simulink model "SCG007C_TC_Development_r01"  (R2017b)
settings: Solver=VariableStepAuto  StartTime=0.0  StopTime=10.0  RelTol=1e-3
values from neighbouring files (symbols this model uses):
  MP_SLIP_val = [ ... (first row only)    [Calibration_r01_v01.m]
  MP_SLIP_x1 = [0.000 0.500 0.750 1.000 1.250 1.500 1.750 2.000 2.500]./2.5.*100    [Calibration_r01_v01.m]
  MP_SLIP_x2 = [0	1	2	3	4	5	6	7	8	9	10	11	12]    [Calibration_r01_v01.m]
  MP_SLIPIP_DSLIP_val = [ ... (first row only)    [Calibration_r01_v01.m]
  MP_SLIPIP_DSLIP_x1 = [0.0 20.0 40.0 60.0 70.0 80.0 90.0 100.0 110.0 120.0 140.0]    [Calibration_r01_v01.m]
  MP_SLIPIP_DSLIP_x2 = [-4.0 -2.0 -1.0 -0.6 0.0 0.1 0.5 3.0 5.0]    [Calibration_r01_v01.m]
  MP_SLIPPP_DSLIP_val = [ ... (first row only)    [Calibration_r01_v01.m]
  MP_SLIPPP_DSLIP_x1 = [0.0 20.0 40.0 60.0 70.0 80.0 90.0 100.0 110.0 120.0 140.0]    [Calibration_r01_v01.m]
  MP_SLIPPP_DSLIP_x2 = [-4.0 -2.0 -1.0 -0.6 0.0 0.1 0.5 3.0 5.0]    [Calibration_r01_v01.m]
undefined symbols (not defined in the file or in its folder): Engine, Standard_Input_Bus, TCS, vicrt_initcallback, vicrt_initmexcallback, vicrt_simulationmanager
libraries: simulink x7, simulink_extras x1
(part 1 of 5)
settings Model: Creator=Stefano.Rapisarda  LastModifiedBy=Stefano.Rapisarda

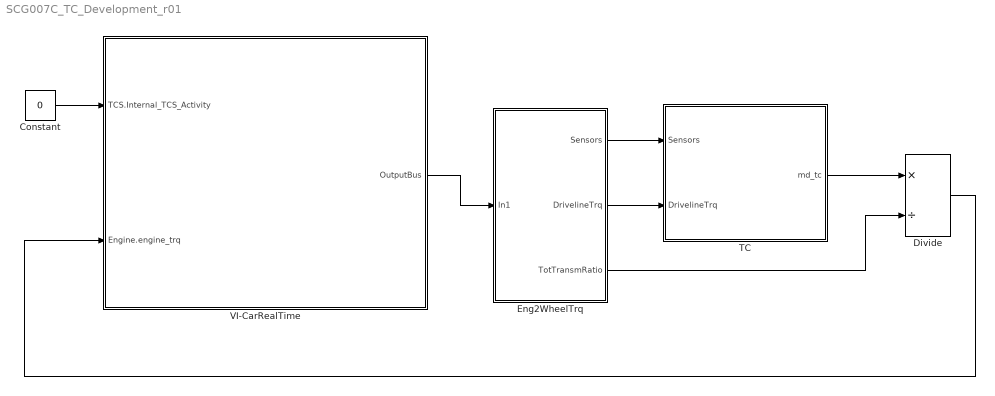
== system SCG007C_TC_Development_r01 ==
  Constant : Constant  Value=0
  Divide : Product  Inputs=*/
  Eng2WheelTrq : Subsystem
  TC : Subsystem
  VI-CarRealTime : Subsystem  InitFcn=vicrt_simulationmanager(0);
      mask help: Full VI-CarRealTime mex integrated with IO Bus
      settings: CopyFcn=set_param(gcb, 'LinkStatus', 'none');  ModelCloseFcn=vicrt_simulationmanager(2);  OpenFcn=vicrt_simulationmanager(1);
      mask Display: image(imread('vehicle.jpg'));color('red');port_label('input',1,'TCS.Internal_TCS_Activity');port_label('input',2,'Engine.engine_trq');port_label('output',1,'OutputBus');
  wires:
  VI-CarRealTime/1(OutputBus) -> Eng2WheelTrq/1(In1)
  TC/1(md_tc) -> Divide/1
  Constant/1 -> VI-CarRealTime/1(TCS.Internal_TCS_Activity)
  Divide/1 -> VI-CarRealTime/2(Engine.engine_trq)
  Eng2WheelTrq/1(Sensors) -> TC/1(Sensors)
  Eng2WheelTrq/2(DrivelineTrq) -> TC/2(DrivelineTrq)
  Eng2WheelTrq/3(TotTransmRatio) -> Divide/2

== system SCG007C_TC_Development_r01/Eng2WheelTrq ==
  In1 : Inport
  Bus Creator : BusCreator  Inputs=2
  Bus Selector : BusSelector  OutputSignals=engine:Max_Engine_torque,engine:Min_engine_torque,transmission:ratio
  Product : Product
  Product1 : Product
  Product2 : Product
  RearDiffRatio : Constant  Value=3.02
  Sensors : Outport
  DrivelineTrq : Outport  Port=2
  TotTransmRatio : Outport  Port=3
  wires:
  In1/1 -> Sensors/1, Bus Selector/1
  Bus Selector/3 -> Product/1  "<transmission:ratio>"
  RearDiffRatio/1 -> Product/2
  Bus Selector/2 -> Product1/1  "<engine:Min_engine_torque>"
  Bus Selector/1 -> Product2/1  "<engine:Max_Engine_torque>"
  Product/1 -> TotTransmRatio/1, Product1/2, Product2/2
  Product2/1 -> Bus Creator/1  "MaxDrivelineTrq"
  Product1/1 -> Bus Creator/2  "MinDrivelineTrq"
  Bus Creator/1 -> DrivelineTrq/1

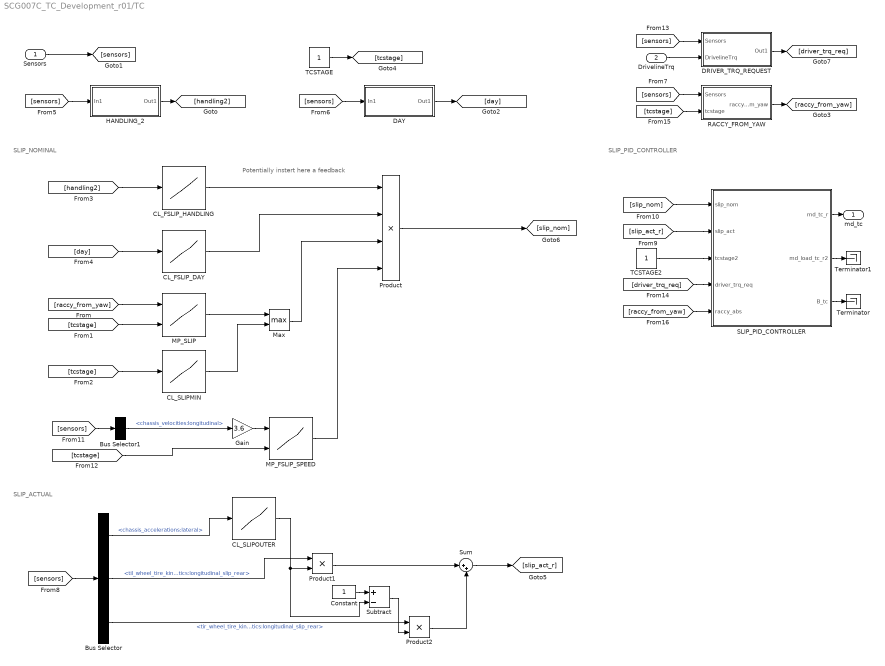
== system SCG007C_TC_Development_r01/TC ==
  note: SLIP_PID_CONTROLLER
  note: Potentially instert here a feedback
  note: SLIP_ACTUAL
  note: SLIP_NOMINAL
  Sensors : Inport
  DrivelineTrq : Inport  Port=2
  Bus Selector : BusSelector  OutputSignals=chassis_accelerations:lateral,til_wheel_tire_kinematics:longitudinal_slip_rear,tir_wheel_tire_kinematics:longitudinal_slip_rear
  Bus Selector1 : BusSelector  OutputSignals=chassis_velocities:longitudinal
  CL_FSLIP_DAY : Lookup_n-D  NumberOfTableDimensions=1  BreakpointsForDimension1=[-1,0,1]  Table=[1,1,1]  InternalRulePriority=Speed  RndMeth=Simplest  InputSameDT=on
  CL_FSLIP_HANDLING : Lookup_n-D  NumberOfTableDimensions=1  BreakpointsForDimension1=[-1,0,1]  Table=[1,1,1]  InternalRulePriority=Speed  RndMeth=Simplest  InputSameDT=on
  CL_SLIPMIN : Lookup_n-D  NumberOfTableDimensions=1  BreakpointsForDimension1=[1,2,3]  Table=[2,2,2]  InternalRulePriority=Speed  RndMeth=Simplest  InputSameDT=on
  CL_SLIPOUTER : Lookup_n-D  NumberOfTableDimensions=1  BreakpointsForDimension1=[-3,-2,-1,0,1,2,3]  Table=[0.8,0.7,0.6,0.5,0.6,0.7,0.8]  InternalRulePriority=Speed  RndMeth=Simplest  InputSameDT=on
  Constant : Constant
  DAY : Subsystem
  DRIVER_TRQ_REQUEST : Subsystem
  Gain : Gain  Gain=3.6
  HANDLING_2 : Subsystem
  MP_FSLIP_SPEED : Lookup_n-D  LookupTableObject=''  BreakpointsForDimension1=[0,500]  BreakpointsForDimension2=[1,2,3]  BreakpointsForDimension1FirstPoint=10  BreakpointsForDimension2FirstPoint=10  BreakpointsForDimension1Spacing=12  BreakpointsForDimension2Spacing=12  IndexSearchMethod=Evenly spaced points  Table=[1 1 1;1 1 1]  InterpMethod=Flat  DiagnosticForOutOfRangeInput=Error  InternalRulePriority=Speed  RndMeth=Simplest  InputSameDT=on
  MP_SLIP : Lookup_n-D  LookupTableObject=''  BreakpointsForDimension1=MP_SLIP_x1  BreakpointsForDimension2=MP_SLIP_x2  BreakpointsForDimension1FirstPoint=10  BreakpointsForDimension2FirstPoint=10  BreakpointsForDimension1Spacing=12  BreakpointsForDimension2Spacing=12  IndexSearchMethod=Evenly spaced points  Table=MP_SLIP_val  InterpMethod=Flat  DiagnosticForOutOfRangeInput=Error  InternalRulePriority=Speed  RndMeth=Simplest  InputSameDT=on
  Max : MinMax  Function=max  Inputs=2
  Product : Product  Inputs=4
  Product1 : Product
  Product2 : Product
  RACCY_FROM_YAW : Subsystem
  SLIP_PID_CONTROLLER : Subsystem
  Subtract : Sum  Inputs=+-
  Sum : Sum  Inputs=|++
  TCSTAGE : Constant
  TCSTAGE2 : Constant
  Terminator : Terminator
  Terminator1 : Terminator
  md_tc : Outport
  wires:
  [raccy_from_yaw] -> MP_SLIP/1
  [tcstage] -> MP_SLIP/2
  [tcstage] -> CL_SLIPMIN/1
  [handling2] -> CL_FSLIP_HANDLING/1
  [day] -> CL_FSLIP_DAY/1
  MP_SLIP/1 -> Max/1
  CL_SLIPMIN/1 -> Max/2
  CL_FSLIP_HANDLING/1 -> Product/1
  CL_FSLIP_DAY/1 -> Product/2
  Max/1 -> Product/3
  Sensors/1 -> [sensors]
  HANDLING_2/1(Out1) -> [handling2]
  [sensors] -> HANDLING_2/1(In1)
  [sensors] -> DAY/1(In1)
  DAY/1(Out1) -> [day]
  [sensors] -> RACCY_FROM_YAW/1(Sensors)
  RACCY_FROM_YAW/1(raccy_from_yaw) -> [raccy_from_yaw]
  TCSTAGE/1 -> [tcstage]
  [sensors] -> Bus Selector/1
  Bus Selector/2 -> Product1/1  "<til_wheel_tire_kinematics:longitudinal_slip_rear>"
  Bus Selector/1 -> CL_SLIPOUTER/1  "<chassis_accelerations:lateral>"
  Constant/1 -> Subtract/1
  CL_SLIPOUTER/1 -> Subtract/2, Product1/2
  Bus Selector/3 -> Product2/1  "<tir_wheel_tire_kinematics:longitudinal_slip_rear>"
  Subtract/1 -> Product2/2
  Product1/1 -> Sum/1
  Product2/1 -> Sum/2
  Sum/1 -> [slip_act_r]
  Product/1 -> [slip_nom]
  [slip_nom] -> SLIP_PID_CONTROLLER/1(slip_nom)
  [slip_act_r] -> SLIP_PID_CONTROLLER/2(slip_act)
  SLIP_PID_CONTROLLER/1(md_tc_r) -> md_tc/1
  MP_FSLIP_SPEED/1 -> Product/4
  [sensors] -> Bus Selector1/1
  Bus Selector1/1 -> Gain/1  "<chassis_velocities:longitudinal>"
  [tcstage] -> MP_FSLIP_SPEED/2
  SLIP_PID_CONTROLLER/3(B_tc) -> Terminator/1
  SLIP_PID_CONTROLLER/2(md_load_tc_r2) -> Terminator1/1
  TCSTAGE2/1 -> SLIP_PID_CONTROLLER/3(tcstage2)
  [sensors] -> DRIVER_TRQ_REQUEST/1(Sensors)
  DRIVER_TRQ_REQUEST/1(Out1) -> [driver_trq_req]
  [driver_trq_req] -> SLIP_PID_CONTROLLER/4(driver_trq_req)
  Gain/1 -> MP_FSLIP_SPEED/1
  [tcstage] -> RACCY_FROM_YAW/2(tcstage)
  DrivelineTrq/1 -> DRIVER_TRQ_REQUEST/2(DrivelineTrq)
  [raccy_from_yaw] -> SLIP_PID_CONTROLLER/5(raccy_abs)

== system SCG007C_TC_Development_r01/VI-CarRealTime ==
  TCS.Internal_TCS_Activity : Inport
  Engine.engine_trq : Inport  Port=2
  Input_Bus : Subsystem  LoadFcn=vicrt_initcallback(gcb);
      settings: CopyFcn=vicrt_initcallback(gcb);
  Output_Bus : Subsystem  Description=Outputs
      settings: CopyFcn=%set_param(gcb, 'LinkStatus', 'none')
  vicrt_mex Standard : Subsystem  mask{vicrt_inputfile='D:\VI-Grade_WD\SCG007C_2\SCG007C_R07_500kW_BaseSetupSiff_Coasting_send_svm.xml', vicrt_outprefix='', intStep=0.001, AniFlag=off, inpPortDim=378, outPortDim=1516, NoDirectFeedthrough=on}
      mask prompts: vicrt_inputfile "VI-CarRealtime input file"; vicrt_outprefix "VI-CarRealTime output prefix"; intStep "Integration step"; AniFlag "live animation"; inpPortDim "input port dimension"; outPortDim "output port dimension"; NoDirectFeedthrough "Direct Feedthrough Off"
      mask init:
      | custDriv=[1,1,1];
      settings: CopyFcn=set_param(gcb, 'LinkStatus', 'none')
  OutputBus : Outport
  wires:
  vicrt_mex Standard/1(Out1) -> Output_Bus/1(Outputs)
  Input_Bus/1(vicrt input) -> vicrt_mex Standard/1(In1)
  TCS.Internal_TCS_Activity/1 -> Input_Bus/1(TCS.Internal_TCS_Activity)
  Engine.engine_trq/1 -> Input_Bus/2(Engine.engine_trq)
  Output_Bus/1(OutputBus) -> OutputBus/1

== system SCG007C_TC_Development_r01/TC/DAY ==
  In1 : Inport
  Constant : Constant  Value=0
  Terminator : Terminator
  Out1 : Outport
  wires:
  Constant/1 -> Out1/1
  In1/1 -> Terminator/1

== system SCG007C_TC_Development_r01/TC/DRIVER_TRQ_REQUEST ==
  Sensors : Inport
  DrivelineTrq : Inport  Port=2
  Add : Sum
  Bus Selector : BusSelector  OutputSignals=engine:Max_Engine_torque,engine:Min_engine_torque,driver_demands:throttle
  Bus Selector1 : BusSelector  OutputSignals=MaxDrivelineTrq,MinDrivelineTrq
  Product : Product
  Subtract : Sum  Inputs=+-
  Terminator : Terminator
  Terminator2 : Terminator
  Out1 : Outport
  wires:
  Sensors/1 -> Bus Selector/1
  Subtract/1 -> Product/1
  Product/1 -> Add/1
  Add/1 -> Out1/1
  Bus Selector/2 -> Terminator/1  "<engine:Min_engine_torque>"
  Bus Selector/3 -> Product/2  "<driver_demands:throttle>"
  Bus Selector/1 -> Terminator2/1  "<engine:Max_Engine_torque>"
  DrivelineTrq/1 -> Bus Selector1/1
  Bus Selector1/1 -> Subtract/1  "<MaxDrivelineTrq>"
  Bus Selector1/2 -> Add/2, Subtract/2  "<MinDrivelineTrq>"

== system SCG007C_TC_Development_r01/TC/HANDLING_2 ==
  In1 : Inport
  Constant : Constant  Value=0
  Terminator : Terminator
  Out1 : Outport
  wires:
  In1/1 -> Terminator/1
  Constant/1 -> Out1/1

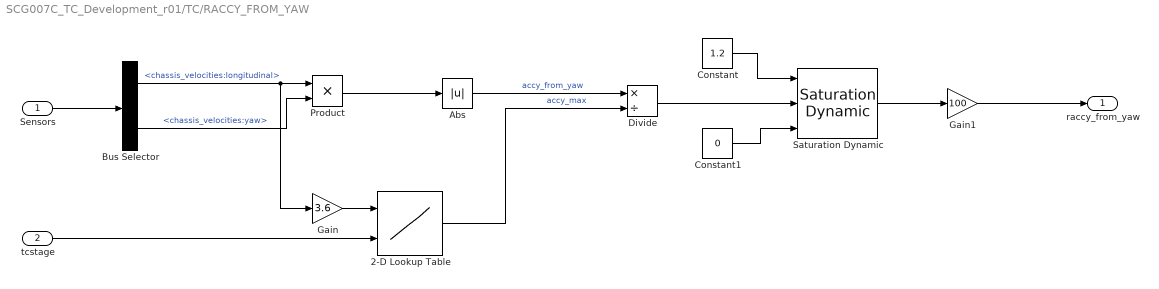
== system SCG007C_TC_Development_r01/TC/RACCY_FROM_YAW ==
  Sensors : Inport
  tcstage : Inport  Port=2
  2-D Lookup Table : Lookup_n-D  BreakpointsForDimension1=[1:3]  BreakpointsForDimension2=[1:3]  InternalRulePriority=Speed  RndMeth=Simplest  InputSameDT=on
  Abs : Abs
  Bus Selector : BusSelector  OutputSignals=chassis_velocities:longitudinal,chassis_velocities:yaw
  Constant : Constant  Value=1.2
  Constant1 : Constant  Value=0
  Divide : Product  Inputs=*/
  Gain : Gain  Gain=3.6
  Gain1 : Gain  Gain=100
  Product : Product
  Saturation Dynamic : simulink/Discontinuities/Saturation Dynamic  OutMin=[]  OutMax=[]  OutDataTypeStr=Inherit: Same as second input  OutDataType=fixdt(1, 16)  OutScaling=2^-10  DoSatur=off
  raccy_from_yaw : Outport
  wires:
  Sensors/1 -> Bus Selector/1
  Bus Selector/1 -> Gain/1, Product/1  "<chassis_velocities:longitudinal>"
  Bus Selector/2 -> Product/2  "<chassis_velocities:yaw>"
  Product/1 -> Abs/1
  Abs/1 -> Divide/1  "accy_from_yaw"
  2-D Lookup Table/1 -> Divide/2  "accy_max"
  Divide/1 -> Saturation Dynamic/2
  Constant/1 -> Saturation Dynamic/1
  Constant1/1 -> Saturation Dynamic/3
  Saturation Dynamic/1 -> Gain1/1
  Gain/1 -> 2-D Lookup Table/1
  tcstage/1 -> 2-D Lookup Table/2
  Gain1/1 -> raccy_from_yaw/1

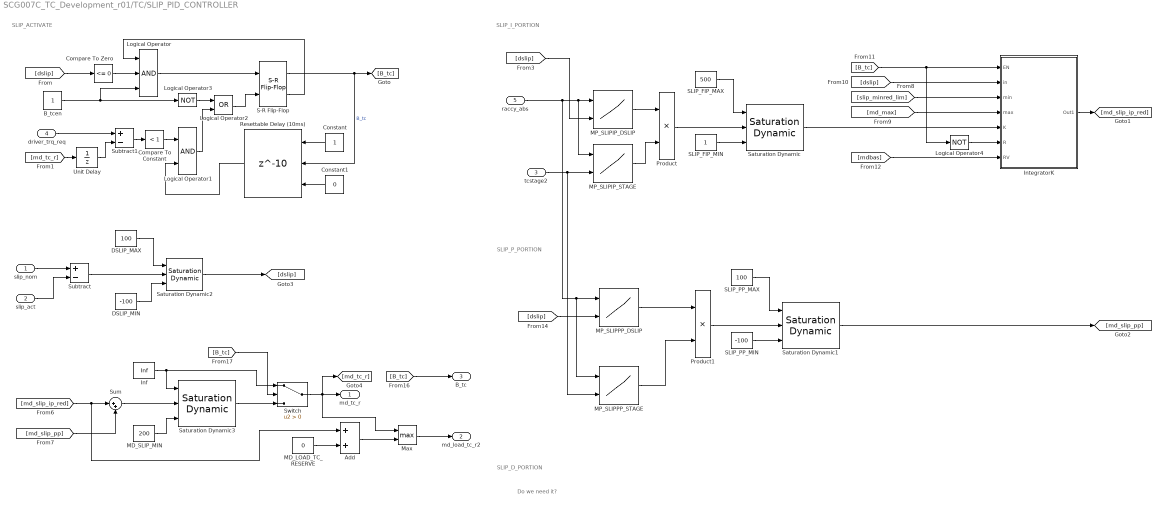
== system SCG007C_TC_Development_r01/TC/SLIP_PID_CONTROLLER ==
  note: Do we need it?
  note: SLIP_I_PORTION
  note: SLIP_ACTIVATE
  note: SLIP_P_PORTION
  note: SLIP_D_PORTION
  slip_nom : Inport
  slip_act : Inport  Port=2
  tcstage2 : Inport  Port=3
  driver_trq_req : Inport  Port=4
  raccy_abs : Inport  Port=5
  Add : Sum
  B_tcen : Constant
  Compare To Constant : simulink/Logic and Bit Operations/Compare To Constant  relop=<  const=1  OutDataTypeStr=boolean
  Compare To Zero : simulink/Logic and Bit Operations/Compare To Zero  relop=<=  OutDataTypeStr=boolean
  Constant : Constant
  Constant1 : Constant  Value=0
  DSLIP_MAX : Constant  Value=100
  DSLIP_MIN : Constant  Value=-100
  Inf : Constant  Value=Inf
  IntegratorK : Subsystem
  Logical Operator : Logic  Inputs=3  AllPortsSameDT=off  OutDataTypeStr=boolean
  Logical Operator1 : Logic  AllPortsSameDT=off  OutDataTypeStr=boolean
  Logical Operator2 : Logic  Operator=OR  AllPortsSameDT=off  OutDataTypeStr=boolean
  Logical Operator3 : Logic  Operator=NOT  AllPortsSameDT=off  OutDataTypeStr=boolean
  Logical Operator4 : Logic  Operator=NOT  AllPortsSameDT=off  OutDataTypeStr=boolean
  MD_LOAD_TC_RESERVE : Constant  Value=0
  MD_SLIP_MIN : Constant  Value=200
  MP_SLIPIP_DSLIP : Lookup_n-D  BreakpointsForDimension1=MP_SLIPIP_DSLIP_x1  BreakpointsForDimension2=MP_SLIPIP_DSLIP_x2  Table=MP_SLIPIP_DSLIP_val  InternalRulePriority=Speed  RndMeth=Simplest  InputSameDT=on
  MP_SLIPIP_STAGE : Lookup_n-D  BreakpointsForDimension1=[0,20,40,60,70,80,90,100,110,120,140]  BreakpointsForDimension2=[0,1]  Table=reshape([1,1,1,1,1,1,1,1,1,1,1,1,1,1,1,1,1,1,1,1,1,1],11,2)  InternalRulePriority=Speed  RndMeth=Simplest  InputSameDT=on
  MP_SLIPPP_DSLIP : Lookup_n-D  BreakpointsForDimension1=MP_SLIPPP_DSLIP_x1  BreakpointsForDimension2=MP_SLIPPP_DSLIP_x2  Table=MP_SLIPPP_DSLIP_val  InternalRulePriority=Speed  RndMeth=Simplest  InputSameDT=on
  MP_SLIPPP_STAGE : Lookup_n-D  BreakpointsForDimension1=[0,20,40,60,70,80,90,100,110,120,140]  BreakpointsForDimension2=[0,1]  Table=reshape([1,1,1,1,1,1,1,1,1,1,1,1,1,1,1,1,1,1,1,1,1,1],11,2)  InternalRulePriority=Speed  RndMeth=Simplest  InputSameDT=on
  Max : MinMax  Function=max  Inputs=2
  Product : Product
  Product1 : Product
  Resettable Delay (10ms) : Delay  DelayLength=10  InitialConditionSource=Input port  ExternalReset=Rising
      settings: InputPortMap=u0,r5,p4
  S-R Flip-Flop : simulink_extras/Flip Flops/S-R Flip-Flop  initial_condition=0
  SLIP_FIP_MAX : Constant  Value=500
  SLIP_FIP_MIN : Constant
  SLIP_PP_MAX : Constant  Value=100
  SLIP_PP_MIN : Constant  Value=-100
  Saturation Dynamic{,1..3} (4 alike) : simulink/Discontinuities/Saturation Dynamic  OutMin=[]  OutMax=[]  OutDataTypeStr=Inherit: Same as second input  OutDataType=fixdt(1, 16)  OutScaling=2^-10  DoSatur=off
  Subtract : Sum  Inputs=+-
  Subtract1 : Sum  Inputs=+-
  Sum : Sum  Inputs=|++
  Switch : Switch  Criteria=u2 > Threshold
  Unit Delay : UnitDelay  SampleTime=-1
  md_tc_r : Outport
  md_load_tc_r2 : Outport  Port=2
  B_tc : Outport  Port=3
  wires:
  [dslip] -> Compare To Zero/1
  Compare To Zero/1 -> Logical Operator/2
  S-R Flip-Flop/2 -> Logical Operator/1
  Logical Operator/1 -> S-R Flip-Flop/1
  B_tcen/1 -> Logical Operator/3, Logical Operator3/1
  Constant/1 -> Resettable Delay (10ms)/1
  Constant1/1 -> Resettable Delay (10ms)/3
  Resettable Delay (10ms)/1 -> Logical Operator1/2
  Logical Operator2/1 -> S-R Flip-Flop/2
  S-R Flip-Flop/1 -> [B_tc], Resettable Delay (10ms)/2  "B_tc"
  Logical Operator3/1 -> Logical Operator2/1
  Logical Operator1/1 -> Logical Operator2/2
  [dslip] -> MP_SLIPIP_DSLIP/2
  MP_SLIPIP_DSLIP/1 -> Product/1
  MP_SLIPIP_STAGE/1 -> Product/2
  Product/1 -> Saturation Dynamic/2
  SLIP_FIP_MAX/1 -> Saturation Dynamic/1
  SLIP_FIP_MIN/1 -> Saturation Dynamic/3
  [md_max] -> IntegratorK/4(max)
  [slip_minred_lim] -> IntegratorK/3(min)
  [dslip] -> IntegratorK/2(in)
  [B_tc] -> Logical Operator4/1, IntegratorK/1(EN)
  Saturation Dynamic/1 -> IntegratorK/5(K)
  Logical Operator4/1 -> IntegratorK/6(R)
  [mdbas] -> IntegratorK/7(RV)
  IntegratorK/1(Out1) -> [md_slip_ip_red]
  raccy_abs/1 -> MP_SLIPPP_STAGE/1, MP_SLIPPP_DSLIP/1, MP_SLIPIP_STAGE/1, MP_SLIPIP_DSLIP/1
  [dslip] -> MP_SLIPPP_DSLIP/2
  tcstage2/1 -> MP_SLIPPP_STAGE/2, MP_SLIPIP_STAGE/2
  MP_SLIPPP_DSLIP/1 -> Product1/1
  MP_SLIPPP_STAGE/1 -> Product1/2
  SLIP_PP_MIN/1 -> Saturation Dynamic1/3
  SLIP_PP_MAX/1 -> Saturation Dynamic1/1
  Product1/1 -> Saturation Dynamic1/2
  Saturation Dynamic1/1 -> [md_slip_pp]
  [B_tc] -> B_tc/1
  Subtract/1 -> Saturation Dynamic2/2
  slip_nom/1 -> Subtract/1
  slip_act/1 -> Subtract/2
  DSLIP_MIN/1 -> Saturation Dynamic2/3
  DSLIP_MAX/1 -> Saturation Dynamic2/1
  Saturation Dynamic2/1 -> [dslip]
  [md_slip_ip_red] -> Add/1, Sum/1
  [md_slip_pp] -> Sum/2
  Sum/1 -> Saturation Dynamic3/2
  MD_SLIP_MIN/1 -> Saturation Dynamic3/3
  Inf/1 -> Switch/1, Saturation Dynamic3/1
  Saturation Dynamic3/1 -> Switch/3
  [B_tc] -> Switch/2
  Switch/1 -> [md_tc_r], Max/1, md_tc_r/1
  Add/1 -> Max/2
  Max/1 -> md_load_tc_r2/1
  MD_LOAD_TC_RESERVE/1 -> Add/2
  [md_tc_r] -> Unit Delay/1
  driver_trq_req/1 -> Subtract1/1
  Unit Delay/1 -> Subtract1/2
  Subtract1/1 -> Compare To Constant/1
  Compare To Constant/1 -> Logical Operator1/1

== system SCG007C_TC_Development_r01/VI-CarRealTime/Input_Bus ==
  TCS.Internal_TCS_Activity : Inport
  Engine.engine_trq : Inport  Port=2
  Bus2Map : Subsystem
  Inputs : Subsystem
  Standard_Input_Bus : Constant
  VicrtBusAssignment : BusAssignment  AssignedSignals=Standard_Input_Bus,TCS.Internal_TCS_Activity,Engine.engine_trq
  vicrt input : Outport
  wires:
  Bus2Map/1(Map Out) -> vicrt input/1
  VicrtBusAssignment/1 -> Bus2Map/1(Bus In)
  Inputs/1(Inputs) -> VicrtBusAssignment/1  "Inputs"
  Standard_Input_Bus/1 -> VicrtBusAssignment/2
  TCS.Internal_TCS_Activity/1 -> VicrtBusAssignment/3
  Engine.engine_trq/1 -> VicrtBusAssignment/4

== system SCG007C_TC_Development_r01/VI-CarRealTime/Output_Bus ==
  Outputs : Inport
  IOmap2bus : Subsystem
  VicrtBusSelector : BusSelector  InitFcn=warning('off','Simulink:blocks:BusSelectorDuplicateLeafSignalInMuxedOutput');  StartFcn=warning('on','Simulink:blocks:BusSelectorDuplicateLeafSignalInMuxedOutput');  OutputSignals=chassis_velocities.longitudinal,condition_sensors.side_slip_angle,til_wheel_tire_kinematics.lateral_slip_front,til_wheel_tire_kinematics.lateral_slip_rear,tir_wheel_tire_kinematics.lateral_slip_front,tir_wheel_tire_kinematics.lateral_slip_rear,til_wheel_tire_kinematics.longitudinal_slip_front,til_wheel_tire_kinematics.longitudinal_slip_rear,tir_wheel_tire_kinematics.longitudinal_slip_front,tir_wheel_tire_kinematics.longitudinal_slip_rear,chassis_accelerations.lateral,chassis_velocities.yaw,engine.Max_Engine_torque,engine.Min_engine_torque,driver_demands.throttle,transmission.ratio,transmission.gear  OutputAsBus=on
  adapter : Subsystem
  OutputBus : Outport
  wires:
  IOmap2bus/1(Out) -> VicrtBusSelector/1
  Outputs/1 -> IOmap2bus/1(In)
  VicrtBusSelector/1 -> adapter/1(inputBus)
  adapter/1(outputBus) -> OutputBus/1

== system SCG007C_TC_Development_r01/VI-CarRealTime/vicrt_mex Standard ==
  In1 : Inport
  vicrt_mex : S-Function  InitFcn=vicrt_initmexcallback(gcb);  FunctionName=vicrt_mex  Parameters=vicrt_inputfile,vicrt_outprefix,AniFlag,intStep,inpPortDim,outPortDim,NoDirectFeedthrough  SFunctionDeploymentMode=off  EnableBusSupport=off
  Out1 : Outport
  wires:
  vicrt_mex/1 -> Out1/1
  In1/1 -> vicrt_mex/1

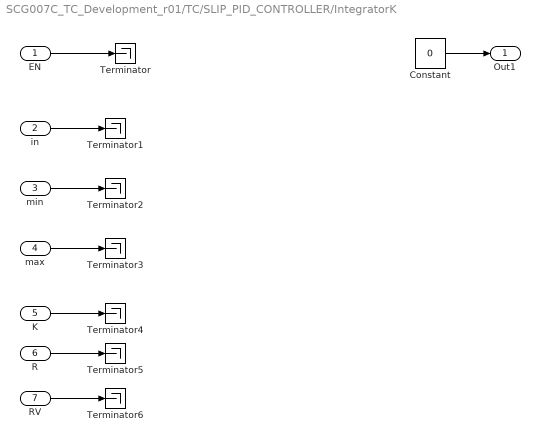
== system SCG007C_TC_Development_r01/TC/SLIP_PID_CONTROLLER/IntegratorK ==
  EN : Inport
  in : Inport  Port=2
  min : Inport  Port=3
  max : Inport  Port=4
  K : Inport  Port=5
  R : Inport  Port=6
  RV : Inport  Port=7
  Constant : Constant  Value=0
  Terminator{,1..6} (7 alike) : Terminator
  Out1 : Outport
  wires:
  EN/1 -> Terminator/1
  in/1 -> Terminator1/1
  min/1 -> Terminator2/1
  max/1 -> Terminator3/1
  K/1 -> Terminator4/1
  R/1 -> Terminator5/1
  RV/1 -> Terminator6/1
  Constant/1 -> Out1/1

== system SCG007C_TC_Development_r01/VI-CarRealTime/Input_Bus/Bus2Map ==
  Bus In : Inport
  Bus Selector : BusSelector  OutputSignals=Driver_Demands.str_swa,Subsystem_Activation.Internal_Steering_Column_Activity,Driver_Demands.rack_displacement,Driver_Demands.throttle,Driver_Demands.gear,Driver_Demands.clutch,Driver_Demands.brake,Driver_Demands.target_speed,Driver_Demands.target_acc,Brake_System_General.brk_mast_cyl_pres,Brake_System_General.brk_bias_front,ABS.Internal_ABS_Activity,ABS.ABS_threshold,Driver_Demands.user_maneuver_ID,Driver_Demands.user_input_steering,Driver_Demands.user_input_throttle,Driver_Demands.user_input_braking,Driver_Demands.user_input_gear,Driver_Demands.user_input_clutch,TCS.Internal_TCS_Activity,TCS.TCS_threshold,Friction.tire_mu.L1,Friction.tire_mu.L2,Friction.tire_mu.R1,Friction.tire_mu.R2,Subsystem_Activation.Internal_Brake_System_Activity.L1,Brake_System.brk_mmag_sign.L1,Brake_System.brk_mmag_unsign.L1,Brake_System.brk_pres.L1,Brake_System.brk_pres_gain.L1,Brake_System.brk_mu.L1,Subsystem_Activation.Internal_Brake_System_Activity.L2,Brake_System.brk_mmag_sign.L2,Brake_System.brk_mmag_unsign.L2,Brake_System.brk_pres.L2,Brake_System.brk_pres_gain.L2,Brake_System.brk_mu.L2,Subsystem_Activation.Internal_Brake_System_Activity.R1,Brake_System.brk_mmag_sign.R1,Brake_System.brk_mmag_unsign.R1,Brake_System.brk_pres.R1,Brake_System.brk_pres_gain.R1,Brake_System.brk_mu.R1,Subsystem_Activation.Internal_Brake_System_Activity.R2,Brake_System.brk_mmag_sign.R2,Brake_System.brk_mmag_unsign.R2,Brake_System.brk_pres.R2,Brake_System.brk_pres_gain.R2,Brake_System.brk_mu.R2,Hook.Fx.rear,Hook.Fy.rear,Hook.Fz.rear,Hook.Mx.rear,Hook.My.rear,Hook.Mz.rear,Rear_Steering_Actuator_disp.str_swa.left,Rear_Steering_Actuator_disp.str_swa.right,Steering.steer_at_spindle.L1,Steering.steer_at_spindle.L2,Steering.steer_at_spindle.R1,Steering.steer_at_spindle.R2,Subsystem_Activation.Internal_Clutch_Activity,Subsystem_Activation.Internal_Engine_Activity,Subsystem_Activation.Internal_Motor_to_Clutch_Activity,Subsystem_Activation.Internal_Motor_to_GearBox_Activity,Subsystem_Activation.Internal_Motor_to_CentralDifferential_Activity,Subsystem_Activation.Internal_Motor_to_FrontDifferential_Activity,Subsystem_Activation.Internal_Motor_to_RearDifferential_Activity,Subsystem_Activation.Internal_Motor_to_FrontRightWheel_Activity,Subsystem_Activation.Internal_Motor_to_FrontLeftWheel_Activity,Subsystem_Activation.Internal_Motor_to_RearRightWheel_Activity,Subsystem_Activation.Internal_Motor_to_RearLeftWheel_Activity,Subsystem_Activation.Internal_Engine_Idle_MaxRev_Controls_Activity,Subsystem_Activation.Internal_Gearbox_Activity,Subsystem_Activation.Internal_CentralDifferential_Activity,Subsystem_Activation.Internal_FrontDifferential_Activity,Subsystem_Activation.Internal_RearDifferential_Activity,Engine.engine_omega,Engine.engine_max_trq,Engine.engine_min_trq,Engine.engine_trq,Engine.clutch_inputplate_torque,Engine.non_termic_engine_trq,Engine.efficiency,Engine.throttle_scaling,Engine.control_mode,Engine.throttle_offset,GearBox.efficiency,GearBox.transmission_ratio,GearBox.diff_central_inputshaft_torque,GearBox.clutch_outputplate_angle,GearBox.clutch_outputplate_omega,GearBox.clutch_outputplate_alpha,GearBox.automatic_gearbox_shifting_mode,Clutch.clutch_trq,Clutch.gearbox_inputshaft_torque,Clutch.inputplate_angle,Clutch.inputplate_omega,Clutch.inputplate_alpha,Clutch.efficiency,Differential_Central.efficiency,Differential_Central.diff_front_inputshaft_torque,Differential_Central.diff_rear_inputshaft_torque,Differential_Central.gearbox_outputshaft_angle,Differential_Central.gearbox_outputshaft_omega,Differential_Central.gearbox_outputshaft_alpha,Differential_Front.efficiency,Differential_Front.wheel_front_left_torque,Differential_Front.wheel_front_right_torque,Differential_Front.diff_central_front_outputshaft_angle,Differential_Front.diff_central_front_outputshaft_omega,Differential_Front.diff_central_front_outputshaft_alpha,Differential_Rear.efficiency,Differential_Rear.wheel_rear_left_torque,Differential_Rear.wheel_rear_right_torque,Differential_Rear.diff_central_rear_outputshaft_angle,Differential_Rear.diff_central_rear_outputshaft_omega,Differential_Rear.diff_central_rear_outputshaft_alpha,Generic_Engine_to_Clutch.regeneration_factor,Generic_Engine_to_Clutch.throttle_scaling,Generic_Engine_to_Clutch.control_mode,Generic_Engine_to_Clutch.throttle_offset,Generic_Engine_to_Clutch.efficiency,Generic_Engine_to_Clutch.engine_torque,Generic_Engine_to_Clutch.engine_max_torque,Generic_Engine_to_Clutch.engine_min_torque,Generic_Engine_to_Gearbox.regeneration_factor,Generic_Engine_to_Gearbox.throttle_scaling,Generic_Engine_to_Gearbox.control_mode,Generic_Engine_to_Gearbox.throttle_offset,Generic_Engine_to_Gearbox.efficiency,Generic_Engine_to_Gearbox.engine_torque,Generic_Engine_to_Gearbox.engine_max_torque,Generic_Engine_to_Gearbox.engine_min_torque,Generic_Engine_to_Central_Differential.reverse_mode,Generic_Engine_to_Central_Differential.regeneration_factor,Generic_Engine_to_Central_Differential.throttle_scaling,Generic_Engine_to_Central_Differential.control_mode,Generic_Engine_to_Central_Differential.throttle_offset,Generic_Engine_to_Central_Differential.efficiency,Generic_Engine_to_Central_Differential.engine_torque,Generic_Engine_to_Central_Differential.engine_max_torque,Generic_Engine_to_Central_Differential.engine_min_torque,Generic_Engine_to_Front_Differential.reverse_mode,Generic_Engine_to_Front_Differential.regeneration_factor,Generic_Engine_to_Front_Differential.throttle_scaling,Generic_Engine_to_Front_Differential.control_mode,Generic_Engine_to_Front_Differential.throttle_offset,Generic_Engine_to_Front_Differential.efficiency,Generic_Engine_to_Front_Differential.engine_torque,Generic_Engine_to_Front_Differential.engine_max_torque,Generic_Engine_to_Front_Differential.engine_min_torque,Generic_Engine_to_Rear_Differential.reverse_mode,Generic_Engine_to_Rear_Differential.regeneration_factor,Generic_Engine_to_Rear_Differential.throttle_scaling,Generic_Engine_to_Rear_Differential.control_mode,Generic_Engine_to_Rear_Differential.throttle_offset,Generic_Engine_to_Rear_Differential.efficiency,Generic_Engine_to_Rear_Differential.engine_torque,Generic_Engine_to_Rear_Differential.engine_max_torque,Generic_Engine_to_Rear_Differential.engine_min_torque,Generic_Engine_to_Front_Right_Wheel.reverse_mode,Generic_Engine_to_Front_Right_Wheel.regeneration_factor,Generic_Engine_to_Front_Right_Wheel.throttle_scaling,Generic_Engine_to_Front_Right_Wheel.control_mode,Generic_Engine_to_Front_Right_Wheel.throttle_offset,Generic_Engine_to_Front_Right_Wheel.efficiency,Generic_Engine_to_Front_Right_Wheel.engine_torque,Generic_Engine_to_Front_Right_Wheel.engine_max_torque,Generic_Engine_to_Front_Right_Wheel.engine_min_torque,Generic_Engine_to_Front_Left_Wheel.reverse_mode,Generic_Engine_to_Front_Left_Wheel.regeneration_factor,Generic_Engine_to_Front_Left_Wheel.throttle_scaling,Generic_Engine_to_Front_Left_Wheel.control_mode,Generic_Engine_to_Front_Left_Wheel.throttle_offset,Generic_Engine_to_Front_Left_Wheel.efficiency,Generic_Engine_to_Front_Left_Wheel.engine_torque,Generic_Engine_to_Front_Left_Wheel.engine_max_torque,Generic_Engine_to_Front_Left_Wheel.engine_min_torque,Generic_Engine_to_Rear_Right_Wheel.reverse_mode,Generic_Engine_to_Rear_Right_Wheel.regeneration_factor,Generic_Engine_to_Rear_Right_Wheel.throttle_scaling,Generic_Engine_to_Rear_Right_Wheel.control_mode,Generic_Engine_to_Rear_Right_Wheel.throttle_offset,Generic_Engine_to_Rear_Right_Wheel.efficiency,Generic_Engine_to_Rear_Right_Wheel.engine_torque,Generic_Engine_to_Rear_Right_Wheel.engine_max_torque,Generic_Engine_to_Rear_Right_Wheel.engine_min_torque,Generic_Engine_to_Rear_Left_Wheel.reverse_mode,Generic_Engine_to_Rear_Left_Wheel.regeneration_factor,Generic_Engine_to_Rear_Left_Wheel.throttle_scaling,Generic_Engine_to_Rear_Left_Wheel.control_mode,Generic_Engine_to_Rear_Left_Wheel.throttle_offset,Generic_Engine_to_Rear_Left_Wheel.efficiency,Generic_Engine_to_Rear_Left_Wheel.engine_torque,Generic_Engine_to_Rear_Left_Wheel.engine_max_torque,Generic_Engine_to_Rear_Left_Wheel.engine_min_torque,Antiroll_Bar.activity_flag.front,Antiroll_Bar.activity_flag.rear,Antiroll_Bar.force.front,Antiroll_Bar.force.rear,Subsystem_Activation.Internal_Aero_Activity,Aerodynamic.my_scaling,Aerodynamic.fx_central_scaling,Aerodynamic.fz_front_scaling,Aerodynamic.fz_rear_scaling,Aerodynamic.fx_front,Aerodynamic.fy_front,Aerodynamic.fz_front,Aerodynamic.fx_rear,Aerodynamic.fy_rear,Aerodynamic.fz_rear,Aerodynamic.fx_center,Aerodynamic.fy_center,Aerodynamic.fz_center,Aerodynamic.mx,Aerodynamic.my,Aerodynamic.mz,Irregularity.road.L1,Irregularity.road.L2,Irregularity.road.R1,Irregularity.road.R2,Main_Damper.force.L1,Main_Damper.activity_flag.L1,Main_Damper.force.L2,Main_Damper.activity_flag.L2,Main_Damper.force.R1,Main_Damper.activity_flag.R1,Main_Damper.force.R2,Main_Damper.activity_flag.R2,Main_Spring.force.L1,Main_Spring.activity_flag.L1,Main_Spring.force.L2,Main_Spring.activity_flag.L2,Main_Spring.force.R1,Main_Spring.activity_flag.R1,Main_Spring.force.R2,Main_Spring.activity_flag.R2,Main_Bumpstop.force.L1,Main_Bumpstop.activity_flag.L1,Main_Bumpstop.force.L2,Main_Bumpstop.activity_flag.L2,Main_Bumpstop.force.R1,Main_Bumpstop.activity_flag.R1,Main_Bumpstop.force.R2,Main_Bumpstop.activity_flag.R2,Main_Reboundstop.force.L1,Main_Reboundstop.activity_flag.L1,Main_Reboundstop.force.L2,Main_Reboundstop.activity_flag.L2,Main_Reboundstop.force.R1,Main_Reboundstop.activity_flag.R1,Main_Reboundstop.force.R2,Main_Reboundstop.activity_flag.R2,Auxiliary_vertical.force.L1,Auxiliary_vertical.activity_flag.L1,Auxiliary_vertical.force.L2,Auxiliary_vertical.activity_flag.L2,Auxiliary_vertical.force.R1,Auxiliary_vertical.activity_flag.R1,Auxiliary_vertical.force.R2,Auxiliary_vertical.activity_flag.R2,Main_Inerter.force.L1,Main_Inerter.activity_flag.L1,Main_Inerter.force.L2,Main_Inerter.activity_flag.L2,Main_Inerter.force.R1,Main_Inerter.activity_flag.R1,Main_Inerter.force.R2,Main_Inerter.activity_flag.R2,Third_Element.Damper_force.front,Third_Element.Damper_activity_flag.front,Third_Element.Damper_force.rear,Third_Element.Damper_activity_flag.rear,Third_Element.Spring.front,Third_Element.Spring_activity_flag.front,Third_Element.Spring.rear,Third_Element.Spring_activity_flag.rear,Mono_Element.Damper.front,Mono_Element.Damper_activity_flag.front,Mono_Element.Damper.rear,Mono_Element.Damper_activity_flag.rear,Mono_Element.Inerter.front,Mono_Element.Inerter_activity_flag.front,Mono_Element.Inerter.rear,Mono_Element.Inerter_activity_flag.rear,Mono_Element.Spring.front,Mono_Element.Spring_activity_flag.front,Mono_Element.Spring.rear,Mono_Element.Spring_activity_flag.rear,Mono_Element.Bumpstop_Spring.front,Mono_Element.Bumpstop_Spring_activity_flag.front,Mono_Element.Bumpstop_Spring.rear,Mono_Element.Bumpstop_Spring_activity_flag.rear,Mono_Element.Reboundstop_Spring.front,Mono_Element.Reboundstop_Spring_activity_flag.front,Mono_Element.Reboundstop_Spring.rear,Mono_Element.Reboundstop_Spring_activity_flag.rear,Mono_Element.Bumpstop_Damper.front,Mono_Element.Bumpstop_Damper_activity_flag.front,Mono_Element.Bumpstop_Damper.rear,Mono_Element.Bumpstop_Damper_activity_flag.rear,Mono_Element.Reboundstop_Damper.front,Mono_Element.Reboundstop_Damper_activity_flag.front,Mono_Element.Reboundstop_Damper.rear,Mono_Element.Reboundstop_Damper_activity_flag.rear,Mono_Element.Roll_Damper.front,Mono_Element.Roll_Damper_activity_flag.front,Mono_Element.Roll_Damper.rear,Mono_Element.Roll_Damper_activity_flag.rear,Subsystem_Activation.Tire_Force_x.L1,Subsystem_Activation.Tire_Force_y.L1,Subsystem_Activation.Tire_Force_z.L1,Subsystem_Activation.Tire_Moment_x.L1,Subsystem_Activation.Tire_Moment_y.L1,Subsystem_Activation.Tire_Moment_z.L1,Tire_Force.Fx.L1,Tire_Force.Fy.L1,Tire_Force.Fz.L1,Tire_Moment.Mx.L1,Tire_Moment.My.L1,Tire_Moment.Mz.L1,Subsystem_Activation.Tire_Force_x.L2,Subsystem_Activation.Tire_Force_y.L2,Subsystem_Activation.Tire_Force_z.L2,Subsystem_Activation.Tire_Moment_x.L2,Subsystem_Activation.Tire_Moment_y.L2,Subsystem_Activation.Tire_Moment_z.L2,Tire_Force.Fx.L2,Tire_Force.Fy.L2,Tire_Force.Fz.L2,Tire_Moment.Mx.L2,Tire_Moment.My.L2,Tire_Moment.Mz.L2,Subsystem_Activation.Tire_Force_x.R1,Subsystem_Activation.Tire_Force_y.R1,Subsystem_Activation.Tire_Force_z.R1,Subsystem_Activation.Tire_Moment_x.R1,Subsystem_Activation.Tire_Moment_y.R1,Subsystem_Activation.Tire_Moment_z.R1,Tire_Force.Fx.R1,Tire_Force.Fy.R1,Tire_Force.Fz.R1,Tire_Moment.Mx.R1,Tire_Moment.My.R1,Tire_Moment.Mz.R1,Subsystem_Activation.Tire_Force_x.R2,Subsystem_Activation.Tire_Force_y.R2,Subsystem_Activation.Tire_Force_z.R2,Subsystem_Activation.Tire_Moment_x.R2,Subsystem_Activation.Tire_Moment_y.R2,Subsystem_Activation.Tire_Moment_z.R2,Tire_Force.Fx.R2,Tire_Force.Fy.R2,Tire_Force.Fz.R2,Tire_Moment.Mx.R2,Tire_Moment.My.R2,Tire_Moment.Mz.R2,Wheel_driving.moment.L1,Wheel_driving.moment.L2,Wheel_driving.moment.R1,Wheel_driving.moment.R2,Ext_Body.force.X,Ext_Body.force.Y,Ext_Body.force.Z,Ext_Body.moment.X,Ext_Body.moment.Y,Ext_Body.moment.Z,Ext_Ground.force.X,Ext_Ground.force.Y,Ext_Ground.force.Z,Ext_Ground.moment.X,Ext_Ground.moment.Y,Ext_Ground.moment.Z,Ext_Tracking.force.X,Ext_Tracking.force.Y,Ext_Tracking.moment.X,Ext_Tracking.moment.Y
  Mux : Mux  Inputs=378
  Map Out : Outport
  wires:
  Mux/1 -> Map Out/1
  Bus In/1 -> Bus Selector/1
  Bus Selector/1 -> Mux/1  "<str_swa>"
  Bus Selector/2 -> Mux/2  "<Internal_Steering_Column_Activity>"
  Bus Selector/3 -> Mux/3  "<rack_displacement>"
  Bus Selector/4 -> Mux/4  "<throttle>"
  Bus Selector/5 -> Mux/5  "<gear>"
  Bus Selector/6 -> Mux/6  "<clutch>"
  Bus Selector/7 -> Mux/7  "<brake>"
  Bus Selector/8 -> Mux/8  "<target_speed>"
  Bus Selector/9 -> Mux/9  "<target_acc>"
  Bus Selector/10 -> Mux/10  "<brk_mast_cyl_pres>"
  Bus Selector/11 -> Mux/11  "<brk_bias_front>"
  Bus Selector/12 -> Mux/12  "<Internal_ABS_Activity>"
  Bus Selector/13 -> Mux/13  "<ABS_threshold>"
  Bus Selector/14 -> Mux/14  "<user_maneuver_ID>"
  Bus Selector/15 -> Mux/15  "<user_input_steering>"
  Bus Selector/16 -> Mux/16  "<user_input_throttle>"
  Bus Selector/17 -> Mux/17  "<user_input_braking>"
  Bus Selector/18 -> Mux/18  "<user_input_gear>"
  Bus Selector/19 -> Mux/19  "<user_input_clutch>"
  Bus Selector/20 -> Mux/20  "<Internal_TCS_Activity>"
  Bus Selector/21 -> Mux/21  "<TCS_threshold>"
  Bus Selector/22 -> Mux/22  "<L1>"
  Bus Selector/23 -> Mux/23  "<L2>"
  Bus Selector/24 -> Mux/24  "<R1>"
  Bus Selector/25 -> Mux/25  "<R2>"
  Bus Selector/26 -> Mux/26  "<L1>"
  Bus Selector/27 -> Mux/27  "<L1>"
  Bus Selector/28 -> Mux/28  "<L1>"
  Bus Selector/29 -> Mux/29  "<L1>"
  Bus Selector/30 -> Mux/30  "<L1>"
  Bus Selector/31 -> Mux/31  "<L1>"
  Bus Selector/32 -> Mux/32  "<L2>"
  Bus Selector/33 -> Mux/33  "<L2>"
  Bus Selector/34 -> Mux/34  "<L2>"
  Bus Selector/35 -> Mux/35  "<L2>"
  Bus Selector/36 -> Mux/36  "<L2>"
  Bus Selector/37 -> Mux/37  "<L2>"
  Bus Selector/38 -> Mux/38  "<R1>"
  Bus Selector/39 -> Mux/39  "<R1>"
  Bus Selector/40 -> Mux/40  "<R1>"
  Bus Selector/41 -> Mux/41  "<R1>"
  Bus Selector/42 -> Mux/42  "<R1>"
  Bus Selector/43 -> Mux/43  "<R1>"
  Bus Selector/44 -> Mux/44  "<R2>"
  Bus Selector/45 -> Mux/45  "<R2>"
  Bus Selector/46 -> Mux/46  "<R2>"
  Bus Selector/47 -> Mux/47  "<R2>"
  Bus Selector/48 -> Mux/48  "<R2>"
  Bus Selector/49 -> Mux/49  "<R2>"
  Bus Selector/50 -> Mux/50  "<rear>"
  Bus Selector/51 -> Mux/51  "<rear>"
  Bus Selector/52 -> Mux/52  "<rear>"
  Bus Selector/53 -> Mux/53  "<rear>"
  Bus Selector/54 -> Mux/54  "<rear>"
  Bus Selector/55 -> Mux/55  "<rear>"
  Bus Selector/56 -> Mux/56  "<left>"
  Bus Selector/57 -> Mux/57  "<right>"
  Bus Selector/58 -> Mux/58  "<L1>"
  Bus Selector/59 -> Mux/59  "<L2>"
  Bus Selector/60 -> Mux/60  "<R1>"
  Bus Selector/61 -> Mux/61  "<R2>"
  Bus Selector/62 -> Mux/62  "<Internal_Clutch_Activity>"
  Bus Selector/63 -> Mux/63  "<Internal_Engine_Activity>"
  Bus Selector/64 -> Mux/64  "<Internal_Motor_to_Clutch_Activity>"
  Bus Selector/65 -> Mux/65  "<Internal_Motor_to_GearBox_Activity>"
  Bus Selector/66 -> Mux/66  "<Internal_Motor_to_CentralDifferential_Activity>"
  Bus Selector/67 -> Mux/67  "<Internal_Motor_to_FrontDifferential_Activity>"
  Bus Selector/68 -> Mux/68  "<Internal_Motor_to_RearDifferential_Activity>"
  Bus Selector/69 -> Mux/69  "<Internal_Motor_to_FrontRightWheel_Activity>"
  Bus Selector/70 -> Mux/70  "<Internal_Motor_to_FrontLeftWheel_Activity>"
  Bus Selector/71 -> Mux/71  "<Internal_Motor_to_RearRightWheel_Activity>"
  Bus Selector/72 -> Mux/72  "<Internal_Motor_to_RearLeftWheel_Activity>"
  Bus Selector/73 -> Mux/73  "<Internal_Engine_Idle_MaxRev_Controls_Activity>"
  Bus Selector/74 -> Mux/74  "<Internal_Gearbox_Activity>"
  Bus Selector/75 -> Mux/75  "<Internal_CentralDifferential_Activity>"
  Bus Selector/76 -> Mux/76  "<Internal_FrontDifferential_Activity>"
  Bus Selector/77 -> Mux/77  "<Internal_RearDifferential_Activity>"
  Bus Selector/78 -> Mux/78  "<engine_omega>"
  Bus Selector/79 -> Mux/79  "<engine_max_trq>"
  Bus Selector/80 -> Mux/80  "<engine_min_trq>"
  Bus Selector/81 -> Mux/81  "<engine_trq>"
  Bus Selector/82 -> Mux/82  "<clutch_inputplate_torque>"
  Bus Selector/83 -> Mux/83  "<non_termic_engine_trq>"
  Bus Selector/84 -> Mux/84  "<efficiency>"
  Bus Selector/85 -> Mux/85  "<throttle_scaling>"
  Bus Selector/86 -> Mux/86  "<control_mode>"
  Bus Selector/87 -> Mux/87  "<throttle_offset>"
  Bus Selector/88 -> Mux/88  "<efficiency>"
  Bus Selector/89 -> Mux/89  "<transmission_ratio>"
  Bus Selector/90 -> Mux/90  "<diff_central_inputshaft_torque>"
  Bus Selector/91 -> Mux/91  "<clutch_outputplate_angle>"
  Bus Selector/92 -> Mux/92  "<clutch_outputplate_omega>"
  Bus Selector/93 -> Mux/93  "<clutch_outputplate_alpha>"
  Bus Selector/94 -> Mux/94  "<automatic_gearbox_shifting_mode>"
  Bus Selector/95 -> Mux/95  "<clutch_trq>"
  Bus Selector/96 -> Mux/96  "<gearbox_inputshaft_torque>"
  Bus Selector/97 -> Mux/97  "<inputplate_angle>"
  Bus Selector/98 -> Mux/98  "<inputplate_omega>"
  Bus Selector/99 -> Mux/99  "<inputplate_alpha>"
  Bus Selector/100 -> Mux/100  "<efficiency>"
  Bus Selector/101 -> Mux/101  "<efficiency>"
  Bus Selector/102 -> Mux/102  "<diff_front_inputshaft_torque>"
  Bus Selector/103 -> Mux/103  "<diff_rear_inputshaft_torque>"
  Bus Selector/104 -> Mux/104  "<gearbox_outputshaft_angle>"
  Bus Selector/105 -> Mux/105  "<gearbox_outputshaft_omega>"
  Bus Selector/106 -> Mux/106  "<gearbox_outputshaft_alpha>"
  Bus Selector/107 -> Mux/107  "<efficiency>"
  Bus Selector/108 -> Mux/108  "<wheel_front_left_torque>"
  Bus Selector/109 -> Mux/109  "<wheel_front_right_torque>"
  Bus Selector/110 -> Mux/110  "<diff_central_front_outputshaft_angle>"
  Bus Selector/111 -> Mux/111  "<diff_central_front_outputshaft_omega>"
  Bus Selector/112 -> Mux/112  "<diff_central_front_outputshaft_alpha>"
  Bus Selector/113 -> Mux/113  "<efficiency>"
  Bus Selector/114 -> Mux/114  "<wheel_rear_left_torque>"
  Bus Selector/115 -> Mux/115  "<wheel_rear_right_torque>"
  Bus Selector/116 -> Mux/116  "<diff_central_rear_outputshaft_angle>"
  Bus Selector/117 -> Mux/117  "<diff_central_rear_outputshaft_omega>"
  Bus Selector/118 -> Mux/118  "<diff_central_rear_outputshaft_alpha>"
  Bus Selector/119 -> Mux/119  "<regeneration_factor>"
  Bus Selector/120 -> Mux/120  "<throttle_scaling>"
  Bus Selector/121 -> Mux/121  "<control_mode>"
  Bus Selector/122 -> Mux/122  "<throttle_offset>"
  Bus Selector/123 -> Mux/123  "<efficiency>"
  Bus Selector/124 -> Mux/124  "<engine_torque>"
  Bus Selector/125 -> Mux/125  "<engine_max_torque>"
  Bus Selector/126 -> Mux/126  "<engine_min_torque>"
  Bus Selector/127 -> Mux/127  "<regeneration_factor>"
  Bus Selector/128 -> Mux/128  "<throttle_scaling>"
  Bus Selector/129 -> Mux/129  "<control_mode>"
  Bus Selector/130 -> Mux/130  "<throttle_offset>"
  Bus Selector/131 -> Mux/131  "<efficiency>"
  Bus Selector/132 -> Mux/132  "<engine_torque>"
  Bus Selector/133 -> Mux/133  "<engine_max_torque>"
  Bus Selector/134 -> Mux/134  "<engine_min_torque>"
  Bus Selector/135 -> Mux/135  "<reverse_mode>"
  Bus Selector/136 -> Mux/136  "<regeneration_factor>"
  Bus Selector/137 -> Mux/137  "<throttle_scaling>"
  Bus Selector/138 -> Mux/138  "<control_mode>"
  Bus Selector/139 -> Mux/139  "<throttle_offset>"
  Bus Selector/140 -> Mux/140  "<efficiency>"
  Bus Selector/141 -> Mux/141  "<engine_torque>"
  Bus Selector/142 -> Mux/142  "<engine_max_torque>"
  Bus Selector/143 -> Mux/143  "<engine_min_torque>"
  Bus Selector/144 -> Mux/144  "<reverse_mode>"
  Bus Selector/145 -> Mux/145  "<regeneration_factor>"
  Bus Selector/146 -> Mux/146  "<throttle_scaling>"
  Bus Selector/147 -> Mux/147  "<control_mode>"
  Bus Selector/148 -> Mux/148  "<throttle_offset>"
  Bus Selector/149 -> Mux/149  "<efficiency>"
  Bus Selector/150 -> Mux/150  "<engine_torque>"
  Bus Selector/151 -> Mux/151  "<engine_max_torque>"
  Bus Selector/152 -> Mux/152  "<engine_min_torque>"
  Bus Selector/153 -> Mux/153  "<reverse_mode>"
  Bus Selector/154 -> Mux/154  "<regeneration_factor>"
  Bus Selector/155 -> Mux/155  "<throttle_scaling>"
  Bus Selector/156 -> Mux/156  "<control_mode>"
  Bus Selector/157 -> Mux/157  "<throttle_offset>"
  Bus Selector/158 -> Mux/158  "<efficiency>"
  Bus Selector/159 -> Mux/159  "<engine_torque>"
  Bus Selector/160 -> Mux/160  "<engine_max_torque>"
  Bus Selector/161 -> Mux/161  "<engine_min_torque>"
  Bus Selector/162 -> Mux/162  "<reverse_mode>"
  Bus Selector/163 -> Mux/163  "<regeneration_factor>"
  Bus Selector/164 -> Mux/164  "<throttle_scaling>"
  Bus Selector/165 -> Mux/165  "<control_mode>"
  Bus Selector/166 -> Mux/166  "<throttle_offset>"
  Bus Selector/167 -> Mux/167  "<efficiency>"
  Bus Selector/168 -> Mux/168  "<engine_torque>"
  Bus Selector/169 -> Mux/169  "<engine_max_torque>"
  Bus Selector/170 -> Mux/170  "<engine_min_torque>"
  Bus Selector/171 -> Mux/171  "<reverse_mode>"
  Bus Selector/172 -> Mux/172  "<regeneration_factor>"
  Bus Selector/173 -> Mux/173  "<throttle_scaling>"
  Bus Selector/174 -> Mux/174  "<control_mode>"
  Bus Selector/175 -> Mux/175  "<throttle_offset>"
  Bus Selector/176 -> Mux/176  "<efficiency>"
  Bus Selector/177 -> Mux/177  "<engine_torque>"
  Bus Selector/178 -> Mux/178  "<engine_max_torque>"
  Bus Selector/179 -> Mux/179  "<engine_min_torque>"
  Bus Selector/180 -> Mux/180  "<reverse_mode>"
  Bus Selector/181 -> Mux/181  "<regeneration_factor>"
  Bus Selector/182 -> Mux/182  "<throttle_scaling>"
  Bus Selector/183 -> Mux/183  "<control_mode>"
  Bus Selector/184 -> Mux/184  "<throttle_offset>"
  Bus Selector/185 -> Mux/185  "<efficiency>"
  Bus Selector/186 -> Mux/186  "<engine_torque>"
  Bus Selector/187 -> Mux/187  "<engine_max_torque>"
  Bus Selector/188 -> Mux/188  "<engine_min_torque>"
  Bus Selector/189 -> Mux/189  "<reverse_mode>"
  Bus Selector/190 -> Mux/190  "<regeneration_factor>"
  Bus Selector/191 -> Mux/191  "<throttle_scaling>"
  Bus Selector/192 -> Mux/192  "<control_mode>"
  Bus Selector/193 -> Mux/193  "<throttle_offset>"
  Bus Selector/194 -> Mux/194  "<efficiency>"
  Bus Selector/195 -> Mux/195  "<engine_torque>"
  Bus Selector/196 -> Mux/196  "<engine_max_torque>"
  Bus Selector/197 -> Mux/197  "<engine_min_torque>"
  Bus Selector/198 -> Mux/198  "<front>"
  Bus Selector/199 -> Mux/199  "<rear>"
  Bus Selector/200 -> Mux/200  "<front>"
  Bus Selector/201 -> Mux/201  "<rear>"
  Bus Selector/202 -> Mux/202  "<Internal_Aero_Activity>"
  Bus Selector/203 -> Mux/203  "<my_scaling>"
  Bus Selector/204 -> Mux/204  "<fx_central_scaling>"
  Bus Selector/205 -> Mux/205  "<fz_front_scaling>"
  Bus Selector/206 -> Mux/206  "<fz_rear_scaling>"
  Bus Selector/207 -> Mux/207  "<fx_front>"
  Bus Selector/208 -> Mux/208  "<fy_front>"
  Bus Selector/209 -> Mux/209  "<fz_front>"
  Bus Selector/210 -> Mux/210  "<fx_rear>"
  Bus Selector/211 -> Mux/211  "<fy_rear>"
  Bus Selector/212 -> Mux/212  "<fz_rear>"
  Bus Selector/213 -> Mux/213  "<fx_center>"
  Bus Selector/214 -> Mux/214  "<fy_center>"
  Bus Selector/215 -> Mux/215  "<fz_center>"
  Bus Selector/216 -> Mux/216  "<mx>"
  Bus Selector/217 -> Mux/217  "<my>"
  Bus Selector/218 -> Mux/218  "<mz>"
  Bus Selector/219 -> Mux/219  "<L1>"
  Bus Selector/220 -> Mux/220  "<L2>"
  Bus Selector/221 -> Mux/221  "<R1>"
  Bus Selector/222 -> Mux/222  "<R2>"
  Bus Selector/223 -> Mux/223  "<L1>"
  Bus Selector/224 -> Mux/224  "<L1>"
  Bus Selector/225 -> Mux/225  "<L2>"
  Bus Selector/226 -> Mux/226  "<L2>"
  Bus Selector/227 -> Mux/227  "<R1>"
  Bus Selector/228 -> Mux/228  "<R1>"
  Bus Selector/229 -> Mux/229  "<R2>"
  Bus Selector/230 -> Mux/230  "<R2>"
  Bus Selector/231 -> Mux/231  "<L1>"
  Bus Selector/232 -> Mux/232  "<L1>"
  Bus Selector/233 -> Mux/233  "<L2>"
  Bus Selector/234 -> Mux/234  "<L2>"
  Bus Selector/235 -> Mux/235  "<R1>"
  Bus Selector/236 -> Mux/236  "<R1>"
  Bus Selector/237 -> Mux/237  "<R2>"
  Bus Selector/238 -> Mux/238  "<R2>"
  Bus Selector/239 -> Mux/239  "<L1>"
  Bus Selector/240 -> Mux/240  "<L1>"
  Bus Selector/241 -> Mux/241  "<L2>"
  Bus Selector/242 -> Mux/242  "<L2>"
  Bus Selector/243 -> Mux/243  "<R1>"
  Bus Selector/244 -> Mux/244  "<R1>"
  Bus Selector/245 -> Mux/245  "<R2>"
  Bus Selector/246 -> Mux/246  "<R2>"
  Bus Selector/247 -> Mux/247  "<L1>"
  Bus Selector/248 -> Mux/248  "<L1>"
  Bus Selector/249 -> Mux/249  "<L2>"
  Bus Selector/250 -> Mux/250  "<L2>"
  Bus Selector/251 -> Mux/251  "<R1>"
  Bus Selector/252 -> Mux/252  "<R1>"
  Bus Selector/253 -> Mux/253  "<R2>"
  Bus Selector/254 -> Mux/254  "<R2>"
  Bus Selector/255 -> Mux/255  "<L1>"
  Bus Selector/256 -> Mux/256  "<L1>"
  Bus Selector/257 -> Mux/257  "<L2>"
  Bus Selector/258 -> Mux/258  "<L2>"
  Bus Selector/259 -> Mux/259  "<R1>"
  Bus Selector/260 -> Mux/260  "<R1>"
  Bus Selector/261 -> Mux/261  "<R2>"
  Bus Selector/262 -> Mux/262  "<R2>"
  Bus Selector/263 -> Mux/263  "<L1>"
  Bus Selector/264 -> Mux/264  "<L1>"
  Bus Selector/265 -> Mux/265  "<L2>"
  Bus Selector/266 -> Mux/266  "<L2>"
  Bus Selector/267 -> Mux/267  "<R1>"
  Bus Selector/268 -> Mux/268  "<R1>"
  Bus Selector/269 -> Mux/269  "<R2>"
  Bus Selector/270 -> Mux/270  "<R2>"
  Bus Selector/271 -> Mux/271  "<front>"
  Bus Selector/272 -> Mux/272  "<front>"
  Bus Selector/273 -> Mux/273  "<rear>"
  Bus Selector/274 -> Mux/274  "<rear>"
  Bus Selector/275 -> Mux/275  "<front>"
  Bus Selector/276 -> Mux/276  "<front>"
  Bus Selector/277 -> Mux/277  "<rear>"
  Bus Selector/278 -> Mux/278  "<rear>"
  Bus Selector/279 -> Mux/279  "<front>"
  Bus Selector/280 -> Mux/280  "<front>"
  Bus Selector/281 -> Mux/281  "<rear>"
  Bus Selector/282 -> Mux/282  "<rear>"
  Bus Selector/283 -> Mux/283  "<front>"
  Bus Selector/284 -> Mux/284  "<front>"
  Bus Selector/285 -> Mux/285  "<rear>"
  Bus Selector/286 -> Mux/286  "<rear>"
  Bus Selector/287 -> Mux/287  "<front>"
  Bus Selector/288 -> Mux/288  "<front>"
  Bus Selector/289 -> Mux/289  "<rear>"
  Bus Selector/290 -> Mux/290  "<rear>"
  Bus Selector/291 -> Mux/291  "<front>"
  Bus Selector/292 -> Mux/292  "<front>"
  Bus Selector/293 -> Mux/293  "<rear>"
  Bus Selector/294 -> Mux/294  "<rear>"
  Bus Selector/295 -> Mux/295  "<front>"
  Bus Selector/296 -> Mux/296  "<front>"
  Bus Selector/297 -> Mux/297  "<rear>"
  Bus Selector/298 -> Mux/298  "<rear>"
  Bus Selector/299 -> Mux/299  "<front>"
  Bus Selector/300 -> Mux/300  "<front>"
  Bus Selector/301 -> Mux/301  "<rear>"
  Bus Selector/302 -> Mux/302  "<rear>"
  Bus Selector/303 -> Mux/303  "<front>"
  Bus Selector/304 -> Mux/304  "<front>"
  Bus Selector/305 -> Mux/305  "<rear>"
  Bus Selector/306 -> Mux/306  "<rear>"
  Bus Selector/307 -> Mux/307  "<front>"
  Bus Selector/308 -> Mux/308  "<front>"
  Bus Selector/309 -> Mux/309  "<rear>"
  Bus Selector/310 -> Mux/310  "<rear>"
  Bus Selector/311 -> Mux/311  "<L1>"
  Bus Selector/312 -> Mux/312  "<L1>"
  Bus Selector/313 -> Mux/313  "<L1>"
  Bus Selector/314 -> Mux/314  "<L1>"
  Bus Selector/315 -> Mux/315  "<L1>"
  Bus Selector/316 -> Mux/316  "<L1>"
  Bus Selector/317 -> Mux/317  "<L1>"
  Bus Selector/318 -> Mux/318  "<L1>"
  Bus Selector/319 -> Mux/319  "<L1>"
  Bus Selector/320 -> Mux/320  "<L1>"
  Bus Selector/321 -> Mux/321  "<L1>"
  Bus Selector/322 -> Mux/322  "<L1>"
  Bus Selector/323 -> Mux/323  "<L2>"
  Bus Selector/324 -> Mux/324  "<L2>"
  Bus Selector/325 -> Mux/325  "<L2>"
  Bus Selector/326 -> Mux/326  "<L2>"
  Bus Selector/327 -> Mux/327  "<L2>"
  Bus Selector/328 -> Mux/328  "<L2>"
  Bus Selector/329 -> Mux/329  "<L2>"
  Bus Selector/330 -> Mux/330  "<L2>"
  Bus Selector/331 -> Mux/331  "<L2>"
  Bus Selector/332 -> Mux/332  "<L2>"
  Bus Selector/333 -> Mux/333  "<L2>"
  Bus Selector/334 -> Mux/334  "<L2>"
  Bus Selector/335 -> Mux/335  "<R1>"
  Bus Selector/336 -> Mux/336  "<R1>"
  Bus Selector/337 -> Mux/337  "<R1>"
  Bus Selector/338 -> Mux/338  "<R1>"
  Bus Selector/339 -> Mux/339  "<R1>"
  Bus Selector/340 -> Mux/340  "<R1>"
  Bus Selector/341 -> Mux/341  "<R1>"
  Bus Selector/342 -> Mux/342  "<R1>"
  Bus Selector/343 -> Mux/343  "<R1>"
  Bus Selector/344 -> Mux/344  "<R1>"
  Bus Selector/345 -> Mux/345  "<R1>"
  Bus Selector/346 -> Mux/346  "<R1>"
  Bus Selector/347 -> Mux/347  "<R2>"
  Bus Selector/348 -> Mux/348  "<R2>"
  Bus Selector/349 -> Mux/349  "<R2>"
  Bus Selector/350 -> Mux/350  "<R2>"
  Bus Selector/351 -> Mux/351  "<R2>"
  Bus Selector/352 -> Mux/352  "<R2>"
  Bus Selector/353 -> Mux/353  "<R2>"
  Bus Selector/354 -> Mux/354  "<R2>"
  Bus Selector/355 -> Mux/355  "<R2>"
  Bus Selector/356 -> Mux/356  "<R2>"
  Bus Selector/357 -> Mux/357  "<R2>"
  Bus Selector/358 -> Mux/358  "<R2>"
  Bus Selector/359 -> Mux/359  "<L1>"
  Bus Selector/360 -> Mux/360  "<L2>"
  Bus Selector/361 -> Mux/361  "<R1>"
  Bus Selector/362 -> Mux/362  "<R2>"
  Bus Selector/363 -> Mux/363  "<X>"
  Bus Selector/364 -> Mux/364  "<Y>"
  Bus Selector/365 -> Mux/365  "<Z>"
  Bus Selector/366 -> Mux/366  "<X>"
  Bus Selector/367 -> Mux/367  "<Y>"
  Bus Selector/368 -> Mux/368  "<Z>"
  Bus Selector/369 -> Mux/369  "<X>"
  Bus Selector/370 -> Mux/370  "<Y>"
  Bus Selector/371 -> Mux/371  "<Z>"
  Bus Selector/372 -> Mux/372  "<X>"
  Bus Selector/373 -> Mux/373  "<Y>"
  Bus Selector/374 -> Mux/374  "<Z>"
  Bus Selector/375 -> Mux/375  "<X>"
  Bus Selector/376 -> Mux/376  "<Y>"
  Bus Selector/377 -> Mux/377  "<X>"
  Bus Selector/378 -> Mux/378  "<Y>"
